simulink model "task2_lab2"  (R2020b)
settings: Solver=VariableStepAuto  StartTime=0  StopTime=1  RelTol=1e-3  EnableMultiTasking=on
settings Model: Creator=JackShen  LastModifiedBy=mluser
settings DataIOCC: LimitDataPoints=on  ReturnWorkspaceOutputs=off
settings OptimizationCC: LifeSpan=inf
settings DebuggingCC: AllowSymbolicDim=off  SFUnexpectedBacktrackingDiag=warning  SFNoUnconditionalDefaultTransitionDiag=warning  SFExecutionAtInitializationDiag=none  ArithmeticOperatorsInVariantConditions=warning
settings ModelReferenceCC: PropagateSignalLabelsOutOfModel=off
settings SFSimCC: SimUseLocalCustomCode=off  CustomCodeUndefinedFunction=UseInterfaceOnly
settings RTWCC: RTWUseLocalCustomCode=off
settings CodeAppCC: StateflowObjectComments=on
settings GRTTargetCC: TargetLangStandard=C89/C90 (ANSI)
settings ConfigComp: CovMetricSettings=dw  CovSaveCumulativeToWorkspaceVar=on  CovSaveSingleToWorkspaceVar=on  CovExternalEMLEnable=off

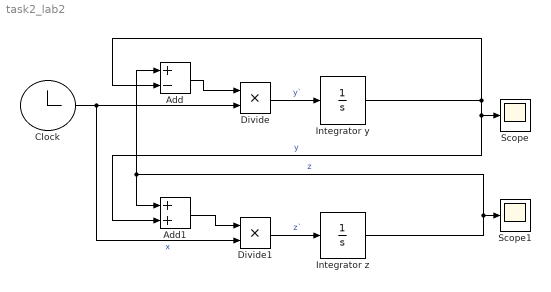
== system task2_lab2 ==
  Add : Sum  Inputs=+-
  Add1 : Sum
  Clock : Clock
  Divide : Product  Inputs=**
  Divide1 : Product  Inputs=**
  Integrator y : Integrator  InitialCondition=1
  Integrator z : Integrator  InitialCondition=1
  Scope : Scope
  Scope1 : Scope
  wires:
  Divide/1 -> Integrator y/1  "y`"
  Divide1/1 -> Integrator z/1  "z`"
  Add/1 -> Divide/1
  Clock/1 -> Divide1/2, Divide/2  "x"
  Integrator y/1 -> Scope/1, Add1/2, Add/2  "y"
  Integrator z/1 -> Add1/1, Add/1, Scope1/1  "z"
  Add1/1 -> Divide1/1
